simulink model "SimulinkVarying"  (R2021b)
settings: Solver=VariableStepAuto  StartTime=0.0  StopTime=160  RelTol=1e-3
libraries: simulink_extras x1, cstblocks x1
settings Model: Creator=raghu  LastModifiedBy=raghu

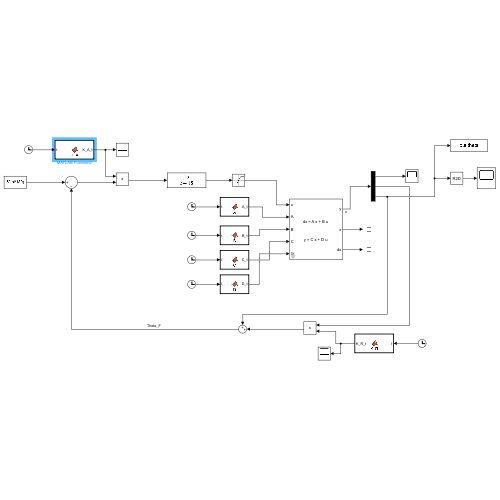
[thumbnail: Simulink's stored preview of the top-level diagram]
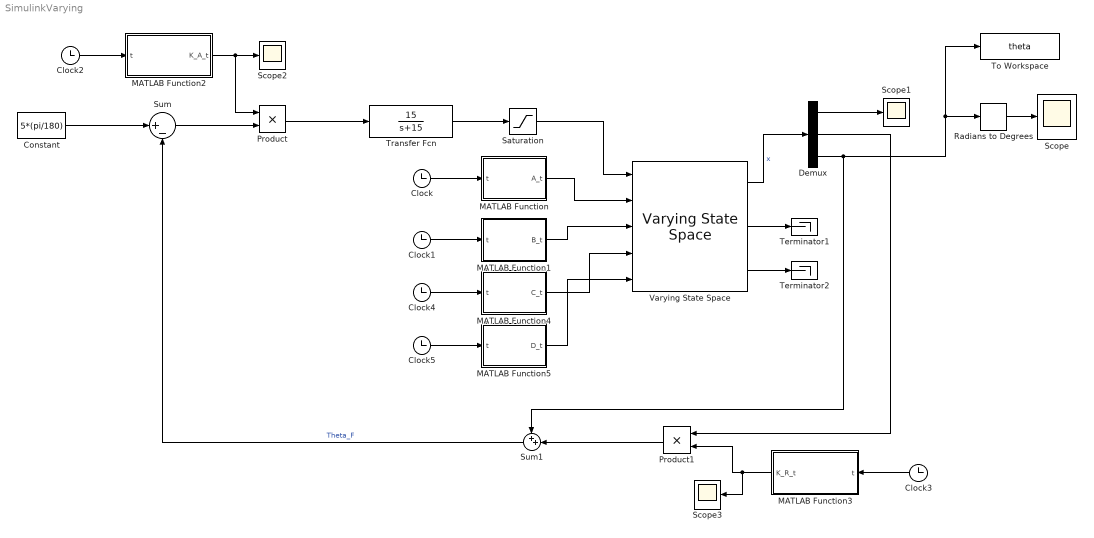
== system SimulinkVarying ==
  Clock{,1..5} (6 alike) : Clock
  Constant : Constant  Value=5*(pi/180)
  Demux : Demux  Outputs=3
  MATLAB Function : MATLAB Function  TreatAsAtomicUnit=on
  MATLAB Function1 : MATLAB Function  TreatAsAtomicUnit=on
  MATLAB Function2 : MATLAB Function  TreatAsAtomicUnit=on
  MATLAB Function3 : MATLAB Function  TreatAsAtomicUnit=on
  MATLAB Function4 : MATLAB Function  TreatAsAtomicUnit=on
  MATLAB Function5 : MATLAB Function  TreatAsAtomicUnit=on
  Product : Product
  Product1 : Product
  Radians to Degrees : simulink_extras/Transformations/Radians to Degrees
  Saturation : Saturate  UpperLimit=10*(pi/180)  LowerLimit=-10*(pi/180)
  Scope{,1..3} (4 alike) : Scope
  Sum : Sum  Inputs=|+-
  Sum1 : Sum  Inputs=++|
  Terminator1 : Terminator
  Terminator2 : Terminator
  To Workspace : ToWorkspace  VariableName=theta  SaveFormat=Timeseries  SampleTime=-1
  Transfer Fcn : TransferFcn  Numerator=[15]  Denominator=[1 15]
  Varying State Space : cstblocks/Linear Parameter Varying/Varying State Space  x0=0  xNames=''  OutputX=on  OutputDX=on
  wires:
  Constant/1 -> Sum/1
  Product1/1 -> Sum1/2
  Transfer Fcn/1 -> Saturation/1
  Sum/1 -> Product/2
  Demux/2 -> Product1/1
  Saturation/1 -> Varying State Space/1
  Sum1/1 -> Sum/2  "Theta_F"
  Demux/1 -> Scope1/1
  Clock/1 -> MATLAB Function/1(t)
  MATLAB Function/1(A_t) -> Varying State Space/2
  MATLAB Function1/1(B_t) -> Varying State Space/3
  Clock1/1 -> MATLAB Function1/1(t)
  Clock2/1 -> MATLAB Function2/1(t)
  MATLAB Function2/1(K_A_t) -> Scope2/1, Product/1
  MATLAB Function3/1(K_R_t) -> Scope3/1, Product1/2
  Varying State Space/3 -> Terminator2/1
  Clock3/1 -> MATLAB Function3/1(t)
  Varying State Space/1 -> Demux/1  "x"
  Varying State Space/2 -> Terminator1/1
  Clock4/1 -> MATLAB Function4/1(t)
  MATLAB Function4/1(C_t) -> Varying State Space/4
  Clock5/1 -> MATLAB Function5/1(t)
  MATLAB Function5/1(D_t) -> Varying State Space/5
  Product/1 -> Transfer Fcn/1
  Demux/3 -> Radians to Degrees/1, To Workspace/1, Sum1/1
  Radians to Degrees/1 -> Scope/1

== matlab function SimulinkVarying/MATLAB Function ==
  data: t input; A_t output
function A_t = A(t)


time =[0 72 152];                %sec

m = [1.20e5 7.38e4 2.44e4];      % Kg;
I_y= [4.41e6 3.28e6 2.03e6];     %Kg-m^2
T_c= [1.37e6 1.52e6 1.58e6];     % N
L_Alpha = [0.001 8.81e5 4.00e4]; % N/rad
l_Alpha = [14.65 10.39 5.67];    % m
l_c= [10.33 9.85 14.26];         % m
U_0= [0.001 984.42 416e3];       % m/sec



pm=polyfit(time,m,2);
m_t=polyval(pm,t);

pI_y=polyfit(time,I_y,2);
I_y_t=polyval(pI_y,t);

pT_c=polyfit(time,T_c,2);
T_c_t=polyval(pT_c,t);

pL_Alpha=polyfit(time,L_Alpha,2);
L_Alpha_t=polyval(pL_Alpha,t);

pl_Alpha=polyfit(time,l_Alpha,2);
l_Alpha_t=polyval(pl_Alpha,t);

pl_c=polyfit(time,l_c,2);
l_c_t=polyval(pl_c,t);

pU_0=polyfit(time,U_0,2);
U_0_t=polyval(pU_0,t);

A_t= [-(L_Alpha_t/(U_0_t)*m_t) U_0_t 0; (L_Alpha_t*l_Alpha_t)/(U_0_t*I_y_t) 0 0;  0 1 0];

== matlab function SimulinkVarying/MATLAB Function2 ==
  data: t input; K_A_t output
function K_A_t = K_A(t)

time=[0 72 152];

K_A=[102.54 52 6.8];

pK_A_1=polyfit([time(1) time(2)], [K_A(1) K_A(2)],1);

pK_A_2=polyfit([time(2) time(3)], [K_A(2) K_A(3)],1);

if t<=time(2)
    K_A_t=polyval(pK_A_1,t);
else
    K_A_t=polyval(pK_A_2,t);
end

== matlab function SimulinkVarying/MATLAB Function3 ==
  data: t input; K_R_t output
function K_R_t = K_R(t)

time =[0 72 152];                %sec

K_R=[0.6 0.6 0.6];

pK_R_1=polyfit([time(1) time(2)],[K_R(1) K_R(2)],1);

pK_R_2=polyfit([time(2) time(3)],[K_R(2) K_R(3)],1);

if t<=time(2)
    K_R_t=polyval(pK_R_1,t);
else
    K_R_t=polyval(pK_R_2,t);
end

== matlab function SimulinkVarying/MATLAB Function4 ==
  data: t input; C_t output
function C_t=C(t)

time=[0 72 152];

C_t = [1 0 0; 0 1 0; 0 0 1];

== matlab function SimulinkVarying/MATLAB Function5 ==
  data: t input; D_t output
function D_t=D(t)

time=[0 72 152];

D_t = [0; 0; 0];

== matlab function SimulinkVarying/MATLAB Function1 ==
  data: t input; B_t output
function B_t = B(t)


time =[0 72 152];                %sec

m = [1.20e5 7.38e4 2.44e4];      % Kg;
I_y= [4.41e6 3.28e6 2.03e6];     %Kg-m^2
T_c= [1.37e6 1.52e6 1.58e6];     % N
L_Alpha = [0.001 8.81e5 4.00e4]; % N/rad
l_Alpha = [14.65 10.39 5.67];    % m
l_c= [10.33 9.85 14.26];         % m
U_0= [0.001 984.42 416e3];       % m/sec



pm=polyfit(time,m,2);
m_t=polyval(pm,t);

pI_y=polyfit(time,I_y,2);
I_y_t=polyval(pI_y,t);

pT_c=polyfit(time,T_c,2);
T_c_t=polyval(pT_c,t);

pL_Alpha=polyfit(time,L_Alpha,2);
L_Alpha_t=polyval(pL_Alpha,t);

pl_Alpha=polyfit(time,l_Alpha,2);
l_Alpha_t=polyval(pl_Alpha,t);

pl_c=polyfit(time,l_c,2);
l_c_t=polyval(pl_c,t);

pU_0=polyfit(time,U_0,2);
U_0_t=polyval(pU_0,t);

B_t= [(T_c_t/m_t); (l_c_t*T_c_t)/I_y_t; 0];
